simulink model "ProjectADRC"  (R2022b)
settings: Solver=ode1  StartTime=0.0  StopTime=6  FixedStep=h  MaxStep=.1  RelTol=1e-6  AbsTol=1e-8  EnableMultiTasking=on
values from neighbouring files (symbols this model uses):
  b = 0.1    [DC_ADRC.m]
  b0 = 40    [DC_ADRC.m]
  J = 0.01    [DC_ADRC.m]
  K = 0.01    [DC_ADRC.m]
  kd = -2.*wc    (= -300)    [DC_ADRC.m]
  kp = wc^2    (= 22500)    [DC_ADRC.m]
  L = 0.5    [DC_ADRC.m]
  R = 1    [DC_ADRC.m]
  wo = 40    [DC_ADRC.m]
libraries: simulink x2
settings Model: Creator=Raj paddy  LastModifiedBy=Raj paddy
settings SolverCC: AutoInsertRateTranBlk=on
settings DataIOCC: SaveFormat=Array  SignalLoggingSaveFormat=ModelDataLogs  SaveOutput=off  ReturnWorkspaceOutputs=off  TimeSaveName=t  SignalLoggingName=sigsOut
settings OptimizationCC: BooleanDataType=off
settings DebuggingCC: SaveWithParameterizedLinksMsg=none  UnderspecifiedInitializationDetection=Classic  MergeDetectMultiDrivingBlocksExec=none  SignalResolutionControl=TryResolveAllWithWarning  MultiTaskDSMMsg=warning  MultiTaskCondExecSysMsg=none  UnconnectedInputMsg=warning  UnconnectedOutputMsg=warning  UnconnectedLineMsg=warning
settings HardwareCC: ProdBitPerPointer=32  ProdBitPerSizeT=32  ProdBitPerPtrDiffT=32  ProdLargestAtomicFloat=None  ProdIntDivRoundTo=Undefined  ProdEndianess=Unspecified  ProdWordSize=32  ProdHWDeviceType=32-bit Generic  TargetUnknown=on
settings ModelReferenceCC: PropagateSignalLabelsOutOfModel=off
settings GRTTargetCC: CombineOutputUpdateFcns=off  GRTInterface=on
settings ConfigComp: CovMetricSettings=dw  CovSaveCumulativeToWorkspaceVar=on  CovSaveSingleToWorkspaceVar=on

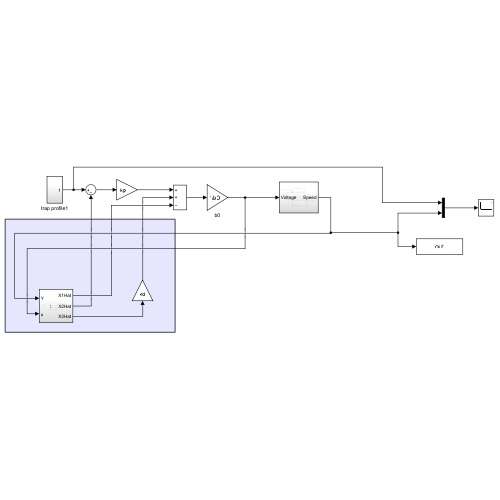
[thumbnail: Simulink's stored preview of the top-level diagram]
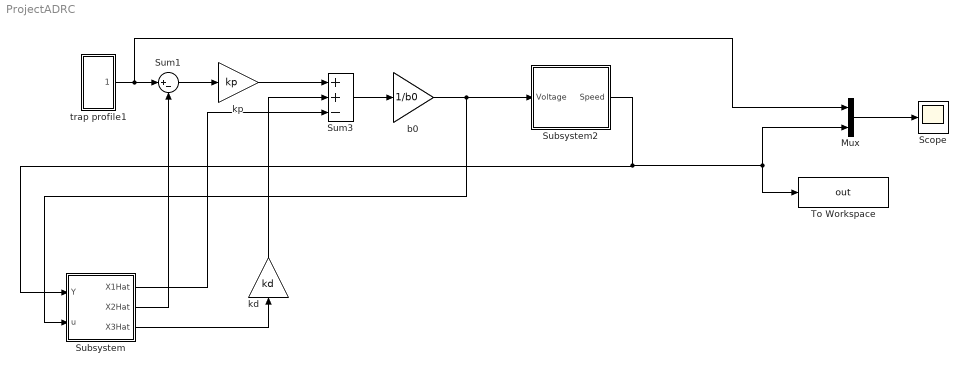
== system ProjectADRC ==
  Mux : Mux  Inputs=2
  Scope : Scope
  Subsystem : Subsystem
  Subsystem2 : Subsystem
  Sum1 : Sum  Inputs=|+-  InputSameDT=on  SaturateOnIntegerOverflow=on  OutDataTypeStr=Inherit: Same as first input
  Sum3 : Sum  Inputs=++-  InputSameDT=on  SaturateOnIntegerOverflow=on  OutDataTypeStr=Inherit: Same as first input
  To Workspace : ToWorkspace  VariableName=out  SaveFormat=Timeseries  SampleTime=-1
  b0 : Gain  Gain=1/b0  SaturateOnIntegerOverflow=on  OutDataTypeStr=Inherit: Same as input  ParamDataTypeStr=Inherit: Same as input
  kd : Gain  Gain=kd  SaturateOnIntegerOverflow=on  OutDataTypeStr=Inherit: Same as input  ParamDataTypeStr=Inherit: Same as input
  kp : Gain  Gain=kp  SaturateOnIntegerOverflow=on  OutDataTypeStr=Inherit: Same as input  ParamDataTypeStr=Inherit: Same as input
  trap profile1 : Subsystem
  wires:
  trap profile1/1(Out1) -> Mux/1, Sum1/1
  Subsystem/2(X2Hat) -> Sum1/2
  Sum3/1 -> b0/1
  Subsystem/1(X1Hat) -> Sum3/3
  b0/1 -> Subsystem/2(u), Subsystem2/1(Voltage)
  kp/1 -> Sum3/1
  kd/1 -> Sum3/2
  Sum1/1 -> kp/1
  Subsystem/3(X3Hat) -> kd/1
  Subsystem2/1(Speed) -> Mux/2, To Workspace/1, Subsystem/1(Y)
  Mux/1 -> Scope/1

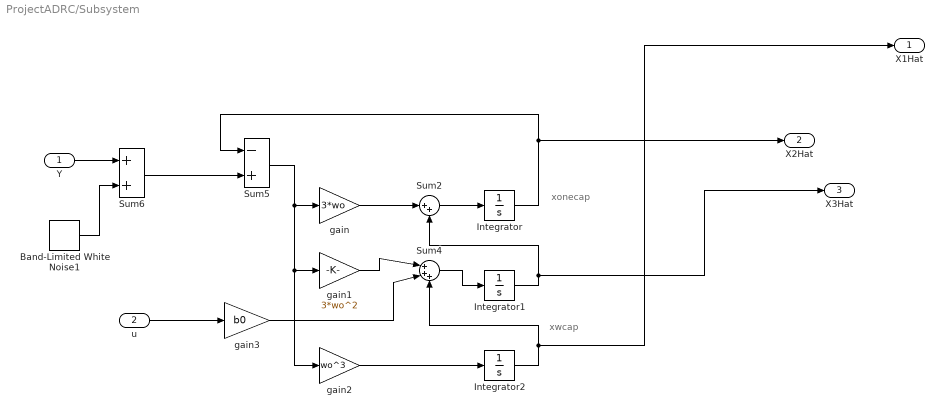
== system ProjectADRC/Subsystem ==
  note: xonecap
  note: xwcap
  Y : Inport
  u : Inport  Port=2
  Band-Limited White Noise1 : simulink/Sources/Band-Limited White Noise  Cov=[1e-9]  Ts=0.001  seed=[23341]
  Integrator : Integrator
  Integrator1 : Integrator
  Integrator2 : Integrator
  Sum2 : Sum  Inputs=|++  InputSameDT=on  SaturateOnIntegerOverflow=on  OutDataTypeStr=Inherit: Same as first input
  Sum4 : Sum  Inputs=|+++  InputSameDT=on  SaturateOnIntegerOverflow=on  OutDataTypeStr=Inherit: Same as first input
  Sum5 : Sum  Inputs=-+  InputSameDT=on  SaturateOnIntegerOverflow=on  OutDataTypeStr=Inherit: Same as first input
  Sum6 : Sum  InputSameDT=on  SaturateOnIntegerOverflow=on  OutDataTypeStr=Inherit: Same as first input
  gain : Gain  Gain=3*wo  SaturateOnIntegerOverflow=on  OutDataTypeStr=Inherit: Same as input  ParamDataTypeStr=Inherit: Same as input
  gain1 : Gain  Gain=3*wo^2  SaturateOnIntegerOverflow=on  OutDataTypeStr=Inherit: Same as input  ParamDataTypeStr=Inherit: Same as input
  gain2 : Gain  Gain=wo^3  SaturateOnIntegerOverflow=on  OutDataTypeStr=Inherit: Same as input  ParamDataTypeStr=Inherit: Same as input
  gain3 : Gain  Gain=b0  SaturateOnIntegerOverflow=on  OutDataTypeStr=Inherit: Same as input  ParamDataTypeStr=Inherit: Same as input
  X1Hat : Outport
  X2Hat : Outport  Port=2
  X3Hat : Outport  Port=3
  wires:
  gain2/1 -> Integrator2/1
  Y/1 -> Sum6/1
  Integrator/1 -> X2Hat/1, Sum5/1
  Sum2/1 -> Integrator/1
  Sum4/1 -> Integrator1/1
  Integrator1/1 -> X3Hat/1, Sum2/2
  Integrator2/1 -> X1Hat/1, Sum4/3
  Sum5/1 -> gain2/1, gain1/1, gain/1
  gain/1 -> Sum2/1
  gain3/1 -> Sum4/2
  gain1/1 -> Sum4/1
  Sum6/1 -> Sum5/2
  Band-Limited White Noise1/1 -> Sum6/2
  u/1 -> gain3/1

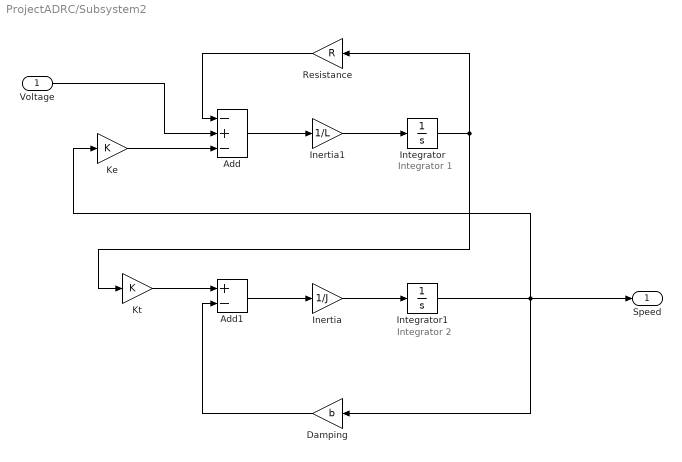
== system ProjectADRC/Subsystem2 ==
  note: Integrator 1
  note: Integrator 2
  Voltage : Inport
  Add : Sum  Inputs=-+-
  Add1 : Sum  Inputs=+-
  Damping : Gain  Gain=b
  Inertia : Gain  Gain=1/J
  Inertia1 : Gain  Gain=1/L
  Integrator : Integrator
  Integrator1 : Integrator
  Ke : Gain  Gain=K
  Kt : Gain  Gain=K
  Resistance : Gain  Gain=R
  Speed : Outport
  wires:
  Inertia1/1 -> Integrator/1
  Inertia/1 -> Integrator1/1
  Add1/1 -> Inertia/1
  Integrator1/1 -> Speed/1, Damping/1, Ke/1
  Add/1 -> Inertia1/1
  Voltage/1 -> Add/2
  Kt/1 -> Add1/1
  Damping/1 -> Add1/2
  Integrator/1 -> Resistance/1, Kt/1
  Resistance/1 -> Add/1
  Ke/1 -> Add/3

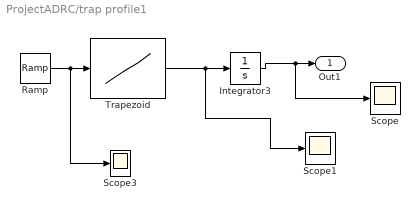
== system ProjectADRC/trap profile1 ==
  Integrator3 : Integrator  LimitOutput=on  UpperSaturationLimit=10  LowerSaturationLimit=0
  Ramp : simulink/Sources/Ramp  slope=1  start=0  InitialOutput=0
  Scope : Scope
  Scope1 : Scope
  Scope3 : Scope
  Trapezoid : Lookup  InputValues=[0 .333333333 .66666666667 1 2]  Table=[0 1.5 1.5 0 0]
  Out1 : Outport
  wires:
  Trapezoid/1 -> Integrator3/1, Scope1/1
  Ramp/1 -> Scope3/1, Trapezoid/1
  Integrator3/1 -> Out1/1, Scope/1
